simulink model "demo_smc_msd"  (R2025a)
settings: Solver=VariableStepAuto  StartTime=0.0  StopTime=3  RelTol=1e-3
settings Model: Creator=xing2  LastModifiedBy=xing2

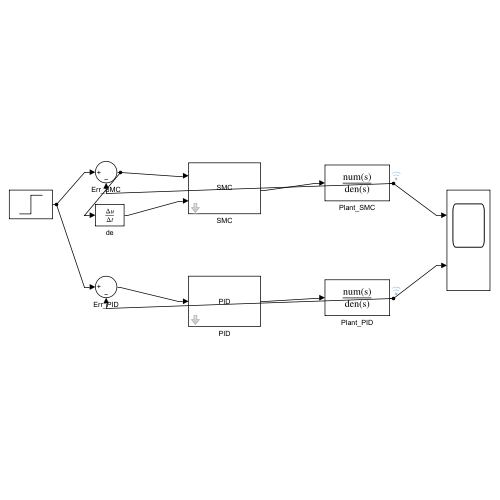
[thumbnail: Simulink's stored preview of the top-level diagram]
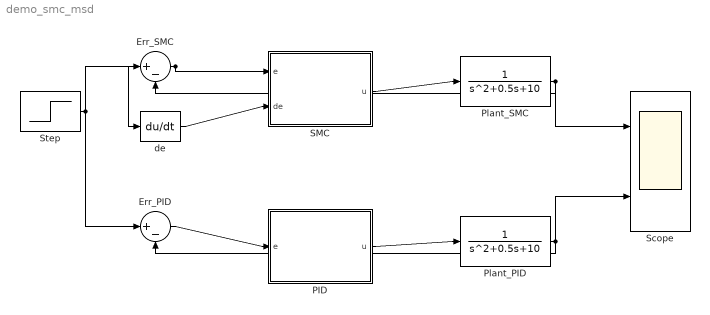
== system demo_smc_msd ==
  Err_PID : Sum  Inputs=|+-
  Err_SMC : Sum  Inputs=|+-
  PID : Subsystem  mask{Kp=50, Ki=20, Kd=5, N=100, UL=10, LL=-10, Kaw=1}
      mask prompts: UL "Upper Limit"; LL "Lower Limit"; Kaw "Anti-Windup Gain"
      mask help: PID Controller with anti-windup and derivative filtering
      mask Display: disp('PID');
  Plant_PID : TransferFcn  Denominator=[1 0.5 10]
  Plant_SMC : TransferFcn  Denominator=[1 0.5 10]
  SMC : Subsystem  mask{lambda=10, K_smc=5, phi=0.1}
      mask prompts: lambda "lambda (slope)"; K_smc "K (gain)"; phi "phi (boundary)"
      mask help: Sliding Mode Controller with boundary layer
      mask Display: disp('SMC');
  Scope : Scope  NumInputPorts=2
  Step : Step  Time=0.5  SampleTime=0
  de : Derivative
  wires:
  Step/1 -> Err_SMC/1, Err_PID/1
  Err_SMC/1 -> SMC/1(e), de/1
  de/1 -> SMC/2(de)
  SMC/1(u) -> Plant_SMC/1
  Plant_SMC/1 -> Scope/1, Err_SMC/2
  Err_PID/1 -> PID/1(e)
  PID/1(u) -> Plant_PID/1
  Plant_PID/1 -> Scope/2, Err_PID/2

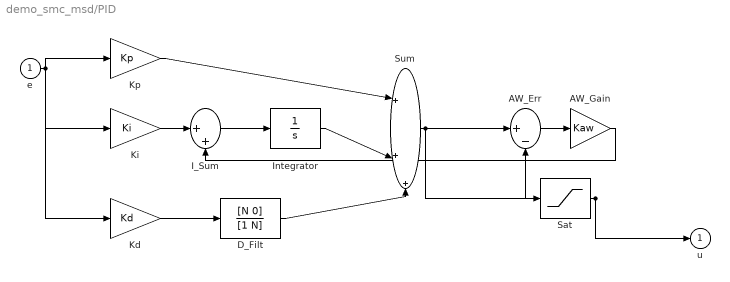
== system demo_smc_msd/PID ==
  e : Inport
  AW_Err : Sum  Inputs=|+-
  AW_Gain : Gain  Gain=Kaw
  D_Filt : TransferFcn  Numerator=[N 0]  Denominator=[1 N]
  I_Sum : Sum  Inputs=|++
  Integrator : Integrator
  Kd : Gain  Gain=Kd
  Ki : Gain  Gain=Ki
  Kp : Gain  Gain=Kp
  Sat : Saturate  UpperLimit=UL  LowerLimit=LL
  Sum : Sum  Inputs=|+++
  u : Outport
  wires:
  AW_Gain/1 -> I_Sum/2
  AW_Err/1 -> AW_Gain/1
  Sat/1 -> AW_Err/2, u/1
  Sum/1 -> AW_Err/1, Sat/1
  D_Filt/1 -> Sum/3
  Integrator/1 -> Sum/2
  Kp/1 -> Sum/1
  Kd/1 -> D_Filt/1
  I_Sum/1 -> Integrator/1
  Ki/1 -> I_Sum/1
  e/1 -> Kd/1, Ki/1, Kp/1

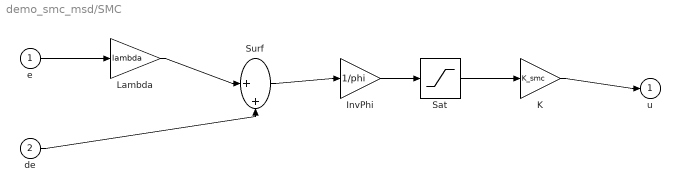
== system demo_smc_msd/SMC ==
  e : Inport
  de : Inport  Port=2
  InvPhi : Gain  Gain=1/phi
  K : Gain  Gain=K_smc
  Lambda : Gain  Gain=lambda
  Sat : Saturate  UpperLimit=1  LowerLimit=-1
  Surf : Sum  Inputs=|++
  u : Outport
  wires:
  K/1 -> u/1
  Sat/1 -> K/1
  InvPhi/1 -> Sat/1
  Surf/1 -> InvPhi/1
  de/1 -> Surf/2
  Lambda/1 -> Surf/1
  e/1 -> Lambda/1
